simulink model "motor_sim"  (R2018a)
settings: Solver=VariableStepAuto  StartTime=0.0  StopTime=10.0  RelTol=1e-3
settings Model: Creator=ABHISHEK  LastModifiedBy=ABHISHEK

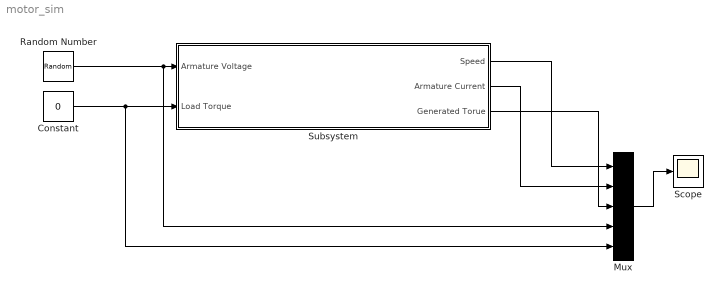
== system motor_sim ==
  Constant : Constant  Value=0
  Mux : Mux  Inputs=5
  Random Number : RandomNumber  SampleTime=0.1
  Scope : Scope
  Subsystem : Subsystem
  wires:
  Mux/1 -> Scope/1
  Subsystem/1("Speed ") -> Mux/1
  Subsystem/2(Armature Current) -> Mux/2
  Subsystem/3("Generated Torue ") -> Mux/3
  Random Number/1 -> Mux/4, Subsystem/1("Armature Voltage ")
  Constant/1 -> Subsystem/2("Load Torque "), Mux/5

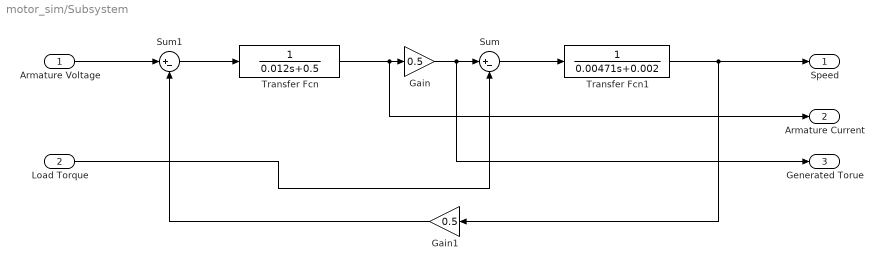
== system motor_sim/Subsystem ==
  "Armature Voltage " : Inport
  "Load Torque " : Inport  Port=2
  Gain : Gain  Gain=0.5
  Gain1 : Gain  Gain=0.5
  Sum : Sum  Inputs=|+-
  Sum1 : Sum  Inputs=|+-
  Transfer Fcn : TransferFcn  Denominator=[0.012 0.5]
  Transfer Fcn1 : TransferFcn  Denominator=[0.00471 0.002]
  "Speed " : Outport
  Armature Current : Outport  Port=2
  "Generated Torue " : Outport  Port=3
  wires:
  Gain1/1 -> Sum1/2
  Transfer Fcn/1 -> Armature Current/1, Gain/1
  Transfer Fcn1/1 -> "Speed "/1, Gain1/1
  "Armature Voltage "/1 -> Sum1/1
  Sum1/1 -> Transfer Fcn/1
  Gain/1 -> "Generated Torue "/1, Sum/1
  Sum/1 -> Transfer Fcn1/1
  "Load Torque "/1 -> Sum/2
